simulink model "AttitudeControlPx4v1_8"  (R2018b)
settings: Solver=VariableStepAuto  StartTime=0.0  StopTime=10.0  RelTol=1e-3
settings Model: Creator=jban039  LastModifiedBy=jeremie

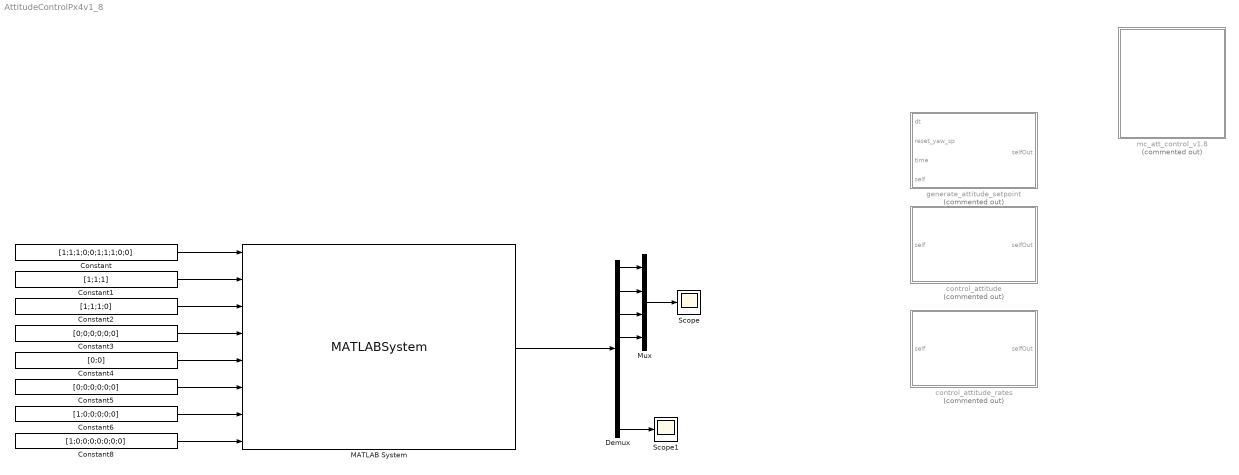
== system AttitudeControlPx4v1_8 ==
  Constant : Constant  Value=[1;1;1;0;0;1;1;1;0;0]
  Constant1 : Constant  Value=[1;1;1]
  Constant2 : Constant  Value=[1;1;1;0]
  Constant3 : Constant  Value=[0;0;0;0;0;0]
  Constant4 : Constant  Value=[0;0]
  Constant5 : Constant  Value=[0;0;0;0;0;0]
  Constant6 : Constant  Value=[1;0;0;0;0;0]
  Constant8 : Constant  Value=[1;0;0;0;0;0;0;0]
  Demux : Demux  Outputs=8
  MATLAB System : MATLABSystem  System=mc_att_control  acro_expo_rp=0.69  acro_expo_y=0.69  acro_pitch_max=720  acro_roll_max=720  acro_superexpo_rp=0.7  acro_superexpo_y=0.7  acro_yaw_max=540  airmode=0  d_term_cutoff_freq=30  pitch_rate_d=0.003  pitch_rate_ff=0  pitch_rate_i=0.05  pitch_rate_max=220  pitch_rate_p=0.15  pitch_p=6.5  pitch_rate_integ_lim=0.3  rattitude_thres=0.8  roll_rate_d=0.003  roll_rate_ff=0  roll_rate_i=0.05  roll_rate_max=220  roll_rate_p=0.15  roll_p=6.5  roll_rate_integ_lim=0.3  tpa_breakpoint_d=1  tpa_breakpoint_i=1  tpa_breakpoint_p=1  tpa_rate_d=0  tpa_rate_i=0  tpa_rate_p=0  yaw_rate_d=0  yaw_rate_ff=0  yaw_rate_i=0.1  yaw_rate_max=200  yaw_rate_p=0.2  yaw_auto_max=45  yaw_p=2.8  yaw_rate_integ_lim=0.3  man_throttle_min=0.08  man_tilt_max_deg=35  yaw_rate_scaling=200  throttle_hover=0.5  throttle_max=1  board_rotation_param=0  board_offset_x=0  board_offset_y=0  board_offset_z=0  bat_scale_en=0  throttle_curve=0  vehicle_status_is_rotary_wing=1  vehicle_status_is_vtol=0  loop_update_rate_hz=250  SimulateUsing=Code generation
      mask Type: mc_att_control
      mask Display:
      | disp(['mc_att_control' char(10) 'v1.8']);
      | port_label('input',1,'v_control_mode_flags');
      | port_label('input',2,'sensor_gyro');
      | port_label('input',3,'manual_control_sp_in');
      | port_label('input',4,'v_rates_sp_in');
      | port_label('input',5,'vehicle_land_detected_in');
      | port_label('input',6,'saturation_status_in');
      | port_label('input',7,'v_att_in');
      | port_label('input',8,'v_att_sp_in');
      | port_label('output',1,'actuators_control');
  Mux : Mux
  Scope : Scope
  Scope1 : Scope
  control_attitude : MATLAB Function  Commented=on  TreatAsAtomicUnit=on
  control_attitude_rates : MATLAB Function  Commented=on  TreatAsAtomicUnit=on
  generate_attitude_setpoint : MATLAB Function  Commented=on  TreatAsAtomicUnit=on
  mc_att_control_v1.8 : Subsystem  Commented=on
  wires:
  Constant/1 -> MATLAB System/1
  Constant8/1 -> MATLAB System/8
  Constant6/1 -> MATLAB System/7
  Constant1/1 -> MATLAB System/2
  Constant2/1 -> MATLAB System/3
  Constant3/1 -> MATLAB System/4
  Constant4/1 -> MATLAB System/5
  Constant5/1 -> MATLAB System/6
  MATLAB System/1 -> Demux/1
  Demux/1 -> Mux/1
  Demux/3 -> Mux/3
  Demux/4 -> Mux/4
  Demux/2 -> Mux/2
  Mux/1 -> Scope/1
  Demux/8 -> Scope1/1

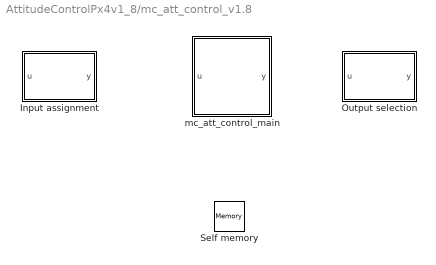
== system AttitudeControlPx4v1_8/mc_att_control_v1.8 ==
  Input assignment : MATLAB Function  TreatAsAtomicUnit=on
  Output selection : MATLAB Function  TreatAsAtomicUnit=on
  Self memory : Memory
  mc_att_control_main : MATLAB Function  TreatAsAtomicUnit=on

== matlab function AttitudeControlPx4v1_8/generate_attitude_setpoint ==
  data: dt input; selfOut output; reset_yaw_sp input; time input; self input
function selfOut =  generate_attitude_setpoint(dt, reset_yaw_sp, time, self)
%GENERATE_ATTITUDE_SETPOINT Generate attitude setpoint (manual control)
%   Based on code from PX4 Firmware (retrieved 2019/01/15, v1.82):
%       https://github.com/PX4/Firmware/blob/master/src/modules/mc_att_control/mc_att_control_main.cpp
%   Written:       J.X.J. Bannwarth, 2019/01/15
%   Last modified: J.X.J. Bannwarth, 2019/01/15

    eul = QuatToEuler( self.v_att.q );
    yaw = eul(3);
    if reset_yaw_sp
        self.man_yaw_sp = yaw;
    elseif ( self.manual_control_sp.z > 0.05 || strcmp( self.airmode, 'roll_pitch_yaw' ) )
        yaw_rate = self.yaw_rate_scaling;
        attitude_setpoint.yaw_sp_move_rate = self.manula_control_sp.r * yaw_rate;
        self.man_yaw_sp = wrap_pi( self.man_yaw_sp + attitude_setpoint.yaw_sp_move_rate*dt );
    end

    % Input mapping for roll & pitch setpoints
    % ----------------------------------------
    % We control the following 2 angles:
    % - tilt angle, given by sqrt(x*x + y*y)
    % - the direction of the maximum tilt in the XY-plane, which also
    % defines the direction of the motion
    %
    % This allows a simple limitation of the tilt angle, the vehicle flies
    % towards the direction that the stick points to, and changes of the
    % stick input are linear.
    x = self.manual_control_sp.x * self.man_tilt_max;
    y = self.manual_control_sp.y * self.man_tilt_max;
    
    % We want to fly towards the direction of (x, y), so we use a
    % perpendicular axis angle vector in the XY-plane
    v = [y, -x];
    v_norm = norm( v );
    
    if (v_norm > self.man_tilt_max) % limit to the configured maximum tilt angle
		v = v * self.man_tilt_max / v_norm;
    end
    
    q_sp_rpy = AxisAngleToQuat( [ v(1); v(2) ] );
    euler_sp = QuatToEuler( q_sp_rpy );
    attitude_setpoint.roll_body  = euler_sp(1);
    attitude_setpoint.pitch_body = euler_sp(2);
    % The axis angle can change the yaw as well (noticeable at higher tilt angles).
	% This is the formula by how much the yaw changes:
	%   let a := tilt angle, b := atan(y/x) (direction of maximum tilt)
	%   yaw = atan(-2 * sin(b) * cos(b) * sin^2(a/2) / (1 - 2 * cos^2(b) * sin^2(a/2))).
    attitude_setpoint.yaw_body = self.man_yaw_sp + euler_sp(3);
    
    if self.vehicle_status.is_vtol
        % Construct attitude setpoint rotation matrix. Modify the setpoints
        % for roll and pitch such that they reflect the user's intention
        % even if a large yaw error (yaw_sp - yaw) is present. In the
        % presence of a yaw error constructing a rotation matrix from the
        % pure euler angle setpoints will lead to unexpected attitude
        % behaviour from the user's view as the euler angle sequence uses
        % the  yaw setpoint and not the current heading of the vehicle.
		% However there's also a coupling effect that causes oscillations
        % for fast roll/pitch changes at higher tilt angles, so we want to
        % avoid using this on multicopters.
		% The effect of that can be seen with:
		% - roll/pitch into one direction, keep it fixed (at high angle)
		% - apply a fast yaw rotation
		% - look at the roll and pitch angles: they should stay pretty much
        % the same as when not yawing
        
        % Calculate our current yaw error
        yaw_error = wrap_pi(attitude_setpoint.yaw_body - yaw);

        % Compute the vector obtained by rotating a z unit vector by the rotation
        % given by the roll and pitch commands of the user
        zB = [0.0; 0.0; 1.0];
        R_sp_roll_pitch = EulerToDcm( [attitude_setpoint.roll_body; attitude_setpoint.pitch_body; 0.0] );
        z_roll_pitch_sp = R_sp_roll_pitch * zB;

        % Transform the vector into a new frame which is rotated around the z axis
        % by the current yaw error. this vector defines the desired tilt when we look
        % into the direction of the desired heading
        R_yaw_correction = EulerToDcm( [0.0; 0.0; -yaw_error] );
        z_roll_pitch_sp = R_yaw_correction * z_roll_pitch_sp;

        % Use the formula z_roll_pitch_sp = R_tilt * [0;0;1]
        % R_tilt is computed from_euler; only true if cos(roll) not equal zero
        % -> valid if roll is not +-pi/2;
        attitude_setpoint.roll_body = -asinf(z_roll_pitch_sp(1));
        attitude_setpoint.pitch_body = atan2f(z_roll_pitch_sp(0), z_roll_pitch_sp(2));
    end
    
    % Publish the setpoint
    q_sp = EulerToQuat( [ attitude_setpoint.roll_body;
                          attitude_setpoint.pitch_body;
                          attitude_setpoint.yaw_body ] );
    attitude_setpoint.q_d = q_sp;
    attitude_setpoint.q_d_valid = true;
    
    attitude_setpoint.thrust_body(3) = -throttle_curve( self.manual_control_sp.z );
    attitude_setpoint.timestamp = time;
end

% Other functions
function throttle = throttle_curve( throttle_stick_input, self )
    switch self.throttle_curve
        case 1 % no rescaling to hover throttle
            throttle = self.man_throttle_min + ...
                throttle_stick_input * (self.throttle_max - self.man_throttle_min);
        otherwise % 0 or other: rescale to hover throttle at 0.5 stick
            if throttle_stick_input < 0.5
                throttle = (self.throttle_hover - self.man_throttle_min) / ...
                    0.5 * throttle_stick_input + self.man_throttle_min;
            else
                throttle = (self.throttle_max - self.throttle_hover) / ...
                    0.5 * (throttle_stick_input - 1.0) + self.throttle_max;
            end
    end
end

% Angle functions
function euler = QuatToEuler( quat )
    euler = DcmToEuler( QuatToDcm( quat ) );
end

function euler = DcmToEuler( dcm )
%DCMTOEULER Convert DCM to Euler angles
%   Based on code from PX4 Firmware:
%       https://github.com/PX4/Matrix/blob/master/matrix/Euler.hpp
%   Written:       J.X.J. Bannwarth, 2019/01/15
%   Last modified: J.X.J. Bannwarth, 2019/01/15
    phi_val   = atan2( dcm(3,2), dcm(3,3) );
    theta_val = asin( -dcm(3,1) );
    psi_val   = atan2( dcm(2,1), dcm(1,1) );
    if abs( theta_val - pi/2 ) < 1e-3
        phi_val = 0;
        psi_val = atan2( dcm(2,3), dcm(1,3) );
    elseif abs( theta_val + pi /2 ) < 1e-3
        phi_val = 0;
        psi_val = atan2( -dcm(2,3), -dcm(1,3) );
    end
    
    euler = [ phi_val; theta_val; psi_val ];
end

function dcm = QuatToDcm( quat )
%DCMTOEULER Convert quaternion to DCM
%   Based on code from PX4 Firmware:
%       https://github.com/PX4/Matrix/blob/master/matrix/Dcm.hpp
%   Written:       J.X.J. Bannwarth, 2019/01/15
%   Last modified: J.X.J. Bannwarth, 2019/01/15
    a = quat(1);
    b = quat(2);
    c = quat(3);
    d = quat(4);
    aa = a * a;
    ab = a * b;
    ac = a * c;
    ad = a * d;
    bb = b * b;
    bc = b * c;
    bd = b * d;
    cc = c * c;
    cd = c * d;
    dd = d * d;

    dcm = zeros(3, 3);
    dcm(1, 1) = aa + bb - cc - dd;
    dcm(1, 2) = 2 * (bc - ad);
    dcm(1, 3) = 2 * (ac + bd);
    dcm(2, 1) = 2 * (bc + ad);
    dcm(2, 2) = aa - bb + cc - dd;
    dcm(2, 3) = 2 * (cd - ab);
    dcm(3, 1) = 2 * (bd - ac);
    dcm(3, 2) = 2 * (ab + cd);
    dcm(3, 3) = aa - bb - cc + dd;
end

function dcm = EulerToDcm( eul )
%EULERTODCM Convert Euler angles to a DCM
%   Based on code from PX4 Firmware:
%       https://github.com/PX4/Matrix/blob/master/matrix/Dcm.hpp
%   Written:       J.X.J. Bannwarth, 2019/01/15
%   Last modified: J.X.J. Bannwarth, 2019/01/15
    phi   = eul(1);
    theta = eul(2);
    psi   = eul(3);
    sinPhi = sin(phi);
    cosPhi = cos(phi);
    cosThe = cos(theta);
    sinThe = sin(theta);
    sinPsi = sin(psi);
    cosPsi = cos(psi);
    
    dcm = zeros(3,3);
    dcm(1,1) = cosThe * cosPsi;
    dcm(1,2) = (sinPhi * sinThe * cosPsi) - (cosPhi * sinPsi);
    dcm(1,3) = (cosPhi * sinThe * cosPsi) + (sinPhi * sinPsi);
    dcm(2,1) = cosThe * sinPsi;
    dcm(2,2) = (sinPhi * sinThe * sinPsi) + (cosPhi * cosPsi);
    dcm(2,3) = (cosPhi * sinThe * sinPsi) - (sinPhi * cosPsi);
    dcm(3,1) = -sinThe;
    dcm(3,2) = sinPhi * cosThe;
    dcm(3,3) = cosPhi * cosThe;
end

function quat = AxisAngleToQuat( axisAngle )
%AXISANGLETOQUAT Convert axis angle representation to quaternion
%   Based on code from PX4 Firmware:
%       https://github.com/PX4/Matrix/blob/master/matrix/Quaternion.hpp
%   axisAngle = [x; y; z]*angle where [x; y; z] is a unit vector
%   Written:       J.X.J. Bannwarth, 2019/01/15
%   Last modified: J.X.J. Bannwarth, 2019/01/15

    angle = norm(axisAngle);
    axis = axisAngle / angle;
    quat = zeros(4,1);
    if (angle < 1e-10)
        quat(1) = 1.0;
        % quat(1) = quat(2) = quat(3) = 0;
    else
        magnitude = sin(angle / 2.0);
        quat(1) = cos(angle / 2.0);
        quat(2) = axis(1) * magnitude;
        quat(3) = axis(2) * magnitude;
        quat(4) = axis(3) * magnitude;
    end
end

function bearing = wrap_pi(bearing)
    % value is inf or NaN
    if (~isfinite(bearing))
        bearing = nan;
        return
    end

    c = 0;

    while (bearing >= 3.14159265)
        bearing = bearing - 6.28318531;

        if (c > 3)
            bearing = nan;
            return
        end
        c = c + 1;
    end

    c = 0;

    while (bearing < -3.14159265)
        bearing = bearing + 6.28318531;

        if (c > 3)
            bearing = nan;
            return
        end
        c = c + 1;
    end
end

== matlab function AttitudeControlPx4v1_8/control_attitude ==
  data: selfOut output; self input
function selfOut =  control_attitude( self )
%CONTROL_ATTITUDE Attitude controller
%   Based on code from PX4 Firmware (retrieved 2019/01/15, v1.82):
%       https://github.com/PX4/Firmware/blob/master/src/modules/mc_att_control/mc_att_control_main.cpp
%   Input: 'vehicle_attitude_setpoint' (depending on mode)
%   Output: self.rates_sp, self.thrust_sp
%   Written:       J.X.J. Bannwarth, 2019/01/15
%   Last modified: J.X.J. Bannwarth, 2019/01/15

    % Physical thrust axis is the negative of body z axis
    self.thrust_sp = -self.v_att_sp.thrust_body(3);

    % Prepare yaw weight from the ratio between roll/pitch and yaw gains
    attitude_gain = self.attitude_p;
    roll_pitch_gain = ( attitude_gain(1) + attitude_gain(2) ) / 2;
    yaw_w = constrain( attitude_gain(3) / roll_pitch_gain, 0, 1 );
    attitude_gain(2) = roll_pitch_gain;

    % Get estimated and desired vehicle attitude
    q  = self.v_att.q;
    qd = self.v_att_sp.q_d;

    % Ensure input quaternions are exactly normalized because
    % acosf(1.00001) == NaN
    q = normalize( q );
    qd = normalize( qd );

    % Calculate reduced desired attitude neglecting vehicle's yaw to
    % prioritize roll and pitch 
    e_z   = QuatToDcmZ( q );
    e_z_d = QuatToDcmZ( qd );
    qd_red = VecsToQuat( e_z, e_z_d );
    
    if ( abs(qd_red(2)) > (1 - 1e-5) ) || ( abs(qd_red(3)) > (1 - 1e-5) )
        % In the infinitesimal corner case where the vehicle and thrust have
        % the completely opposite direction, full attitude control anyways
        % generates no yaw input and directly takes the combination of roll
        % and pitch leading to the correct desired yaw. Ignoring this case
        % would still be totally safe and stable.
        qd_red = qd;
    else
        % Transform rotation from current to desired thrust vector into a
        % world frame reduced desired attitude
        qd_red = qd_red * q;
    end
    
    % Mix full and reduced desired attitude
    q_mix = QuatMult( InvertQuat(qd_red), qd );
    q_mix = q_mix * SignNoZero( q_mix(1) );
    
    % Catch numerical problems with the domain of acosf and asinf
    q_mix(1) = constrain( q_mix(1), -1, 1 );
    q_mix(4) = constrain( q_mix(4), -1, 1 );
    qd = qd_red * [ cos( yaw_w * acos(q_mix(1)) );
                    0;
                    0;
                    sin( yaw_w * asin(q_mix(4)) ) ];

    % Quaternion attitude control law, qe is rotation from q to qd
    qe = QuatMult( InvertQuat(q), qd );

    % Using sin(alpha/2) scaled rotation axis as attitude error (see
    % quaternion definition by axis angle)
    % Also taking care of the antipodal unit quaternion ambiguity
    % qe(2:4) corresponds to the imaginary part of the quaternion
    eq = 2 .* SignNoZero(qe(1)) .* qe(2:4);

    % calculate angular rates setpoint
    self.rates_sp = eq .* attitude_gain;

    % Feed forward the yaw setpoint rate.
    % yaw_sp_move_rate is the feed forward commanded rotation around the
    % world z-axis, but we need to apply it in the body frame (because
    % self.rates_sp is expressed in the body frame).
    % Therefore we infer the world z-axis (expressed in the body frame) by
    % taking the last column of R.transposed (== q.inversed) and multiply
    % it by the yaw setpoint rate (yaw_sp_move_rate).
    % This yields a vector representing the commanded rotation around the
    % world z-axis expressed in the body frame such that it can be added to
    % the rates setpoint.
    self.rates_sp = self.rates_sp + QuatToDcmZ( InvertQuat(q) ) * self.v_att_sp.yaw_sp_move_rate;
    
    % limit rates
    for i = 1:3
        if (( self.v_control_mode.flag_control_velocity_enabled || ...
                self.v_control_mode.flag_control_auto_enabled ) && ...
                ~self.v_control_mode.flag_control_manual_enabled )
            self.rates_sp(i) = constrain(self.rates_sp(i), -self.auto_rate_max(i), self.auto_rate_max(i));
        else
            self.rates_sp(i) = constrain(self.rates_sp(i), -self.mc_rate_max(i), self.mc_rate_max(i));
        end
    end
end

% Other functions
function out = normalize( in )
    out = in ./ norm(in);
end

function y = constrain( x, x_min, x_max )
    y = max( min(x, x_max), x_min );
end

function out = SignNoZero( in )
%SIGNNOZERO SIGNUM function that returns 1 at 0
%   Based on code from PX4 Firmware:
%       https://github.com/PX4/Firmware/blob/master/src/lib/mathlib/math/Functions.hpp
%   Written:       J.X.J. Bannwarth, 2019/01/15
%   Last modified: J.X.J. Bannwarth, 2019/01/17
    out = ( 0 <= in ) - ( in < 0 );
end

% Angle functions
function euler = QuatToEuler( quat )
    euler = DcmToEuler( QuatToDcm( quat ) );
end

function euler = DcmToEuler( dcm )
%DCMTOEULER Convert DCM to Euler angles
%   Based on code from PX4 Firmware:
%       https://github.com/PX4/Matrix/blob/master/matrix/Euler.hpp
%   Written:       J.X.J. Bannwarth, 2019/01/15
%   Last modified: J.X.J. Bannwarth, 2019/01/15
    phi_val   = atan2( dcm(3,2), dcm(3,3) );
    theta_val = asin( -dcm(3,1) );
    psi_val   = atan2( dcm(2,1), dcm(1,1) );
    if abs( theta_val - pi/2 ) < 1e-3
        phi_val = 0;
        psi_val = atan2( dcm(2,3), dcm(1,3) );
    elseif abs( theta_val + pi /2 ) < 1e-3
        phi_val = 0;
        psi_val = atan2( -dcm(2,3), -dcm(1,3) );
    end
    
    euler = [ phi_val; theta_val; psi_val ];
end

function dcm = QuatToDcm( quat )
%QUATTODCM Convert quaternion to DCM
%   Based on code from PX4 Firmware:
%       https://github.com/PX4/Matrix/blob/master/matrix/Dcm.hpp
%   Written:       J.X.J. Bannwarth, 2019/01/15
%   Last modified: J.X.J. Bannwarth, 2019/01/15
    a = quat(1);
    b = quat(2);
    c = quat(3);
    d = quat(4);
    aa = a * a;
    ab = a * b;
    ac = a * c;
    ad = a * d;
    bb = b * b;
    bc = b * c;
    bd = b * d;
    cc = c * c;
    cd = c * d;
    dd = d * d;

    dcm = zeros(3, 3);
    dcm(1, 1) = aa + bb - cc - dd;
    dcm(1, 2) = 2 * (bc - ad);
    dcm(1, 3) = 2 * (ac + bd);
    dcm(2, 1) = 2 * (bc + ad);
    dcm(2, 2) = aa - bb + cc - dd;
    dcm(2, 3) = 2 * (cd - ab);
    dcm(3, 1) = 2 * (bd - ac);
    dcm(3, 2) = 2 * (ab + cd);
    dcm(3, 3) = aa - bb - cc + dd;
end

function dcmZ = QuatToDcmZ( quat )
%QUATTODCMZ Convert quaternion to corresponding body z-axis
%	Last orthogonal unit basis vector
%   == last column of the equivalent rotation matrix
%   but calculated more efficiently than a full conversion
%   Based on code from PX4 Firmware:
%       https://github.com/PX4/Matrix/blob/master/matrix/Dcm.hpp
%   Written:       J.X.J. Bannwarth, 2019/01/15
%   Last modified: J.X.J. Bannwarth, 2019/01/15

    a = quat(1);
    b = quat(2);
    c = quat(3);
    d = quat(4);
    dcmZ = [ 2 * (a * c + b * d);
             2 * (c * d - a * b);
             a * a - b * b - c * c + d * d ];
end

function dcm = EulerToDcm( eul )
%EULERTODCM Convert Euler angles to a DCM
%   Based on code from PX4 Firmware:
%       https://github.com/PX4/Matrix/blob/master/matrix/Dcm.hpp
%   Written:       J.X.J. Bannwarth, 2019/01/15
%   Last modified: J.X.J. Bannwarth, 2019/01/15
    phi   = eul(1);
    theta = eul(2);
    psi   = eul(3);
    sinPhi = sin(phi);
    cosPhi = cos(phi);
    cosThe = cos(theta);
    sinThe = sin(theta);
    sinPsi = sin(psi);
    cosPsi = cos(psi);
    
    dcm = zeros(3,3);
    dcm(1,1) = cosThe * cosPsi;
    dcm(1,2) = (sinPhi * sinThe * cosPsi) - (cosPhi * sinPsi);
    dcm(1,3) = (cosPhi * sinThe * cosPsi) + (sinPhi * sinPsi);
    dcm(2,1) = cosThe * sinPsi;
    dcm(2,2) = (sinPhi * sinThe * sinPsi) + (cosPhi * cosPsi);
    dcm(2,3) = (cosPhi * sinThe * sinPsi) - (sinPhi * cosPsi);
    dcm(3,1) = -sinThe;
    dcm(3,2) = sinPhi * cosThe;
    dcm(3,3) = cosPhi * cosThe;
end

function quat = AxisAngleToQuat( axisAngle )
%AXISANGLETOQUAT Convert axis angle representation to quaternion
%   axisAngle = [x; y; z]*angle where [x; y; z] is a unit vector
%   Based on code from PX4 Firmware:
%       https://github.com/PX4/Matrix/blob/master/matrix/Quaternion.hpp
%   Written:       J.X.J. Bannwarth, 2019/01/15
%   Last modified: J.X.J. Bannwarth, 2019/01/15

    angle = norm(axisAngle);
    axis = axisAngle / angle;
    quat = zeros(4,1);
    if (angle < 1e-10)
        quat(1) = 1.0;
        % quat(1) = quat(2) = quat(3) = 0;
    else
        magnitude = sin(angle / 2.0);
        quat(1) = cos(angle / 2.0);
        quat(2) = axis(1) * magnitude;
        quat(3) = axis(2) * magnitude;
        quat(4) = axis(3) * magnitude;
    end
end

function quat = VecsToQuat( src, dst )
%VECSTOQUAT Quaternion from two vectors
%   Generates shortest rotation from source to destination vector
%   Based on code from PX4 Firmware:
%       https://github.com/PX4/Matrix/blob/master/matrix/Quaternion.hpp
%   Written:       J.X.J. Bannwarth, 2019/01/15
%   Last modified: J.X.J. Bannwarth, 2019/01/15
    cr = cross(src, dst);
    dt = dot(src, dst);
    quat = zeros(4,1);
    locEps = 1e-5; % Don't use eps as it's a reserved variable in MATLAB
    if (norm(cr) < locEps && dt < 0)
        % Handle corner cases with 180 degree rotations
        % If the two vectors are parallel, cross product is zero
        % If they point opposite, the dot product is negative
        cr = abs(src);
        if (cr(1) < cr(2))
            if (cr(1) < cr(3))
                cr = [1; 0; 0];
            else
                cr = [0; 0; 1];
            end
        else
            if (cr(2) < cr(3))
                cr = [0; 1; 0];
            else
                cr = [0; 0; 1];
            end
        end
        quat(1) = 0;
        cr = cross(src, cr);
    else
        % Normal case, do half-way quaternion solution
        quat(1) = dt + sqrt( norm(src)^2 * norm(dst)^2 );
    end
    quat(2) = cr(1);
    quat(3) = cr(2);
    quat(4) = cr(3);
    quat = normalize( quat );
end

function quatInv = InvertQuat( quat )
%INVERTQUAT Invert quaternion
%   Based on code from PX4 Firmware:
%       https://github.com/PX4/Matrix/blob/master/matrix/Quaternion.hpp
%   Written:       J.X.J. Bannwarth, 2019/01/15
%   Last modified: J.X.J. Bannwarth, 2019/01/15
    normSq = dot( quat, quat );
    quatInv = ( quat .* [1;-1;-1;-1] ./ normSq );
end

function quatOut = QuatMult( q1, q2 )
%QUATMULT Multiply quaternion q1 by quaternion q2
%   Based on code from PX4 Firmware:
%       https://github.com/PX4/Matrix/blob/master/matrix/Quaternion.hpp
%   Written by:    J.X.J. Bannwarth, 2017/03/28
%   Last modified: J.X.J. Bannwarth, 2017/01/15
    quatOut = [ q1(1) * q2(1) - q1(2) * q2(2) - q1(3) * q2(3) - q1(4) * q2(4) ;
                q1(1) * q2(2) + q1(2) * q2(1) + q1(3) * q2(4) - q1(4) * q2(3) ;
                q1(1) * q2(3) - q1(2) * q2(4) + q1(3) * q2(1) + q1(4) * q2(2) ;
                q1(1) * q2(4) + q1(2) * q2(3) - q1(3) * q2(2) + q1(4) * q2(1) ];
end

function bearing = wrap_pi(bearing)
    % value is inf or NaN
    if (~isfinite(bearing))
        bearing = nan;
        return
    end

    c = 0;

    while (bearing >= 3.14159265)
        bearing = bearing - 6.28318531;

        if (c > 3)
            bearing = nan;
            return
        end
        c = c + 1;
    end

    c = 0;

    while (bearing < -3.14159265)
        bearing = bearing + 6.28318531;

        if (c > 3)
            bearing = nan;
            return
        end
        c = c + 1;
    end
end

== matlab function AttitudeControlPx4v1_8/control_attitude_rates ==
  data: selfOut output; self input
function selfOut =  control_attitude_rates( self )
%CONTROL_ATTITUDE_RATES Attitude rates controller
%   Based on code from PX4 Firmware (retrieved 2019/01/15, v1.82):
%       https://github.com/PX4/Firmware/blob/master/src/modules/mc_att_control/mc_att_control_main.cpp
%   Input: self.rates_sp, self.thrust_sp
%   Output: self.att_control
%   Written:       J.X.J. Bannwarth, 2019/01/15
%   Last modified: J.X.J. Bannwarth, 2019/01/16

    % Reset integral if disarmed */
    if (~self.v_control_mode.flag_armed || self.vehicle_status.is_rotary_wing)
        self.rates_int = zeros(3,1);
    end

    % Get the raw gyro data and correct for thermal errors
    % Note: the original code applies different correction based on which
    % gyro is being used, but since this is a simulation we do not need to
    % worry about this.
    rates = zeros(3,1);
    rates(1) = self.sensor_gyro.x;
    rates(2) = self.sensor_gyro.y;
    rates(3) = self.sensor_gyro.z;

    % Rotate corrected measurements from sensor to body frame
    rates = self.board_rotation * rates;

    % Correct for in-run bias errors
    rates(1) = rates(1) - self.sensor_bias.gyro_x_bias;
    rates(2) = rates(2) - self.sensor_bias.gyro_y_bias;
    rates(3) = rates(3) - self.sensor_bias.gyro_z_bias;

    rates_p_scaled = self.rate_p .* pid_attenuations(self.tpa_breakpoint_p, self.tpa_rate_p, self.thrust_sp);
    rates_i_scaled = self.rate_i .* pid_attenuations(self.tpa_breakpoint_i, self.tpa_rate_i, self.thrust_sp);
    rates_d_scaled = self.rate_d .* pid_attenuations(self.tpa_breakpoint_d, self.tpa_rate_d, self.thrust_sp);

    % Angular rates error
    rates_err = self.rates_sp - rates;

    % Apply low-pass filtering to the rates for D-term
    [ rates_filtered, self.lp_filters_d ] = LowPassFilter2pVector3Apply( rates, self.lp_filters_d );

    self.att_control = rates_p_scaled .* rates_err + ...
        self.rates_int - ...
        rates_d_scaled .* (rates_filtered - self.rates_prev_filtered) / dt + ...
        self.rate_ff .* self.rates_sp;

    self.rates_prev = rates;
    self.rates_prev_filtered = rates_filtered;

    % update integral only if we are not landed */
    if (~self.vehicle_land_detected.maybe_landed && ~self.vehicle_land_detected.landed)
        for i = 1:3
            % Check for positive control saturation
            positive_saturation = ...
                ((i == 1) && self.saturation_status.flags.roll_pos) || ...
                ((i == 2) && self.saturation_status.flags.pitch_pos) || ...
                ((i == 3) && self.saturation_status.flags.yaw_pos);

            % Check for negative control saturation
            negative_saturation = ...
                ((i == 1) && self.saturation_status.flags.roll_neg) || ...
                ((i == 2) && self.saturation_status.flags.pitch_neg) || ...
                ((i == 3) && self.saturation_status.flags.yaw_neg);

            % prevent further positive control saturation
            if (positive_saturation)
                rates_err(i) = min( [rates_err(i), 0.0] );
            end

            % prevent further negative control saturation
            if (negative_saturation)
                rates_err(i) = max( [rates_err(i), 0.0] );
            end

            % Perform the integration using a first order method and do not propagate the result if out of range or invalid
            rate_i = self.rates_int(i) + rates_i_scaled(i) * rates_err(i) * dt;

            if (isfinite(rate_i) && (rate_i > -self.rate_int_lim(i)) && (rate_i < self.rate_int_lim(i)))
                self.rates_int(i) = rate_i;
            end
        end
    end

    % explicitly limit the integrator state */
    for i = 1:3
        self.rates_int(i) = constrain(self.rates_int(i), -self.rate_int_lim(i), self.rate_int_lim(i));
    end

end

% Other functions
function out = normalize( in )
    out = in ./ norm(in);
end

function y = constrain( x, x_min, x_max )
    y = max( min(x, x_max), x_min );
end

function out = SignNoZero( in )
%SIGNNOZERO SIGNUM function that returns 1 at 0
%   Based on code from PX4 Firmware:
%       https://github.com/PX4/Firmware/blob/master/src/lib/mathlib/math/Functions.hpp
%   Written:       J.X.J. Bannwarth, 2019/01/15
%   Last modified: J.X.J. Bannwarth, 2019/01/17
    out = ( 0 <= in ) - ( in < 0 );
end

function pidAttenuationPerAxis = pid_attenuations( tpa_breakpoint, tpa_rate, thrust_sp )
%PID_ATTENUATIONS Throttle PID attenuation
%   Function visualization available here https://www.desmos.com/calculator/gn4mfoddje
%   Input: tpa_breakpoint, tpa_rate, self.thrust_sp
%   Based on code from PX4 Firmware:
%       https://github.com/PX4/Firmware/blob/master/src/modules/mc_att_control/mc_att_control_main.cpp
%   Written:       J.X.J. Bannwarth, 2019/01/16
%   Last modified: J.X.J. Bannwarth, 2019/01/16
    TPA_RATE_LOWER_LIMIT = 0.05;
    tpa = 1.0 - tpa_rate * (abs(thrust_sp) - tpa_breakpoint) / (1.0 - tpa_breakpoint);
    tpa = max([TPA_RATE_LOWER_LIMIT, min([1.0, tpa])]);
    pidAttenuationPerAxis = [ tpa; tpa; 1.0 ];
end

% Lowpass
function [ output, filter ] = LowPassFilter2pVector3Apply( sample, filter )
%LOWPASSFILTER2PVECTOR3APPLY Apply low pass filter
%   Based on code from PX4 Firmware:
%       https://github.com/PX4/Firmware/blob/master/src/lib/mathlib/math/filter/LowPassFilter2pVector3f.hpp
%   Written:       J.X.J. Bannwarth, 2019/01/16
%   Last modified: J.X.J. Bannwarth, 2019/01/16
    delay_element_0 = sample - filter.delay_element_1.*filter.a1 - filter.delay_element_2.*filter.a2;
    output = delay_element_0.*filter.b0 + filter.delay_element_1.*filter.b1 + filter.delay_element_2*filter.b2;
    filter.delay_element_2 = filter.delay_element_1;
    filter.delay_element_1 = delay_element_0;
end

function filter = LowPassFilter2pVectorSetCutOffFrequency( sample_freq, cutoff_freq, filter )
%LOWPASSFILTER2PVECTOR3SETCUTOFFFREQUENCY Set cutoff frequency
%   Based on code from PX4 Firmware:
%       https://github.com/PX4/Firmware/blob/master/src/lib/mathlib/math/filter/LowPassFilter2pVector3f.cpp
%   Written:       J.X.J. Bannwarth, 2019/01/16
%   Last modified: J.X.J. Bannwarth, 2019/01/16
    filter.cutoff_freq = cutoff_freq;

    % Reset delay elements on filter change
    filter.delay_element_1 = zeros(3,1);
    filter.delay_element_2 = zeros(3,1);

    if (filter.cutoff_freq <= 0.0)
        % No filtering
        filter.b0 = 1.0;
        filter.b1 = 0.0;
        filter.b2 = 0.0;

        filter.a1 = 0.0;
        filter.a2 = 0.0;
        return
    end

    fr = sample_freq / filter.cutoff_freq;
    ohm = tanf( pi / fr);
    c = 1.0 + 2.0 * cosf( pi / 4.0) * ohm + ohm * ohm;

    filter.b0 = ohm * ohm / c;
    filter.b1 = 2.0 * filter.b0;
    filter.b2 = filter.b0;

    filter.a1 = 2.0 * (ohm * ohm - 1.0) / c;
    filter.a2 = (1.0 - 2.0 * cosf(pi / 4.0) * ohm + ohm * ohm) / c;
end

function [ output, filter ] = LowPassFilter2pVectorReset( sample, filter )
%LOWPASSFILTER2PVECTOR3SETCUTOFFFREQUENCY Set cutoff frequency
%   Based on code from PX4 Firmware:
%       https://github.com/PX4/Firmware/blob/master/src/lib/mathlib/math/filter/LowPassFilter2pVector3f.cpp
%   Written:       J.X.J. Bannwarth, 2019/01/16
%   Last modified: J.X.J. Bannwarth, 2019/01/16
    dval = sample ./ (filter.b0 + filter.b1 + filter.b2);

    if (isfinite( dval(1) ) && isfinite( dval(2) ) && isfinite( dval(3) ))
        filter.delay_element_1 = dval;
        filter.delay_element_2 = dval;
    else
        filter.delay_element_1 = sample;
        filter.delay_element_2 = sample;
    end

    [ output, filter ] = LowPassFilter2pVector3Apply( sample, filter );
end

% Angle functions  
function euler = QuatToEuler( quat )
    euler = DcmToEuler( QuatToDcm( quat ) );
end

function euler = DcmToEuler( dcm )
%DCMTOEULER Convert DCM to Euler angles
%   Based on code from PX4 Firmware:
%       https://github.com/PX4/Matrix/blob/master/matrix/Euler.hpp
%   Written:       J.X.J. Bannwarth, 2019/01/15
%   Last modified: J.X.J. Bannwarth, 2019/01/15
    phi_val   = atan2( dcm(3,2), dcm(3,3) );
    theta_val = asin( -dcm(3,1) );
    psi_val   = atan2( dcm(2,1), dcm(1,1) );
    if abs( theta_val - pi/2 ) < 1e-3
        phi_val = 0;
        psi_val = atan2( dcm(2,3), dcm(1,3) );
    elseif abs( theta_val + pi /2 ) < 1e-3
        phi_val = 0;
        psi_val = atan2( -dcm(2,3), -dcm(1,3) );
    end
    
    euler = [ phi_val; theta_val; psi_val ];
end

function dcm = QuatToDcm( quat )
%QUATTODCM Convert quaternion to DCM
%   Based on code from PX4 Firmware:
%       https://github.com/PX4/Matrix/blob/master/matrix/Dcm.hpp
%   Written:       J.X.J. Bannwarth, 2019/01/15
%   Last modified: J.X.J. Bannwarth, 2019/01/15
    a = quat(1);
    b = quat(2);
    c = quat(3);
    d = quat(4);
    aa = a * a;
    ab = a * b;
    ac = a * c;
    ad = a * d;
    bb = b * b;
    bc = b * c;
    bd = b * d;
    cc = c * c;
    cd = c * d;
    dd = d * d;

    dcm = zeros(3, 3);
    dcm(1, 1) = aa + bb - cc - dd;
    dcm(1, 2) = 2 * (bc - ad);
    dcm(1, 3) = 2 * (ac + bd);
    dcm(2, 1) = 2 * (bc + ad);
    dcm(2, 2) = aa - bb + cc - dd;
    dcm(2, 3) = 2 * (cd - ab);
    dcm(3, 1) = 2 * (bd - ac);
    dcm(3, 2) = 2 * (ab + cd);
    dcm(3, 3) = aa - bb - cc + dd;
end

function dcmZ = QuatToDcmZ( quat )
%QUATTODCMZ Convert quaternion to corresponding body z-axis
%	Last orthogonal unit basis vector
%   == last column of the equivalent rotation matrix
%   but calculated more efficiently than a full conversion
%   Based on code from PX4 Firmware:
%       https://github.com/PX4/Matrix/blob/master/matrix/Dcm.hpp
%   Written:       J.X.J. Bannwarth, 2019/01/15
%   Last modified: J.X.J. Bannwarth, 2019/01/15

    a = quat(1);
    b = quat(2);
    c = quat(3);
    d = quat(4);
    dcmZ = [ 2 * (a * c + b * d);
             2 * (c * d - a * b);
             a * a - b * b - c * c + d * d ];
end

function dcm = EulerToDcm( eul )
%EULERTODCM Convert Euler angles to a DCM
%   Based on code from PX4 Firmware:
%       https://github.com/PX4/Matrix/blob/master/matrix/Dcm.hpp
%   Written:       J.X.J. Bannwarth, 2019/01/15
%   Last modified: J.X.J. Bannwarth, 2019/01/15
    phi   = eul(1);
    theta = eul(2);
    psi   = eul(3);
    sinPhi = sin(phi);
    cosPhi = cos(phi);
    cosThe = cos(theta);
    sinThe = sin(theta);
    sinPsi = sin(psi);
    cosPsi = cos(psi);
    
    dcm = zeros(3,3);
    dcm(1,1) = cosThe * cosPsi;
    dcm(1,2) = (sinPhi * sinThe * cosPsi) - (cosPhi * sinPsi);
    dcm(1,3) = (cosPhi * sinThe * cosPsi) + (sinPhi * sinPsi);
    dcm(2,1) = cosThe * sinPsi;
    dcm(2,2) = (sinPhi * sinThe * sinPsi) + (cosPhi * cosPsi);
    dcm(2,3) = (cosPhi * sinThe * sinPsi) - (sinPhi * cosPsi);
    dcm(3,1) = -sinThe;
    dcm(3,2) = sinPhi * cosThe;
    dcm(3,3) = cosPhi * cosThe;
end

function quat = AxisAngleToQuat( axisAngle )
%AXISANGLETOQUAT Convert axis angle representation to quaternion
%   axisAngle = [x; y; z]*angle where [x; y; z] is a unit vector
%   Based on code from PX4 Firmware:
%       https://github.com/PX4/Matrix/blob/master/matrix/Quaternion.hpp
%   Written:       J.X.J. Bannwarth, 2019/01/15
%   Last modified: J.X.J. Bannwarth, 2019/01/15

    angle = norm(axisAngle);
    axis = axisAngle / angle;
    quat = zeros(4,1);
    if (angle < 1e-10)
        quat(1) = 1.0;
        % quat(1) = quat(2) = quat(3) = 0;
    else
        magnitude = sin(angle / 2.0);
        quat(1) = cos(angle / 2.0);
        quat(2) = axis(1) * magnitude;
        quat(3) = axis(2) * magnitude;
        quat(4) = axis(3) * magnitude;
    end
end

function quat = VecsToQuat( src, dst )
%VECSTOQUAT Quaternion from two vectors
%   Generates shortest rotation from source to destination vector
%   Based on code from PX4 Firmware:
%       https://github.com/PX4/Matrix/blob/master/matrix/Quaternion.hpp
%   Written:       J.X.J. Bannwarth, 2019/01/15
%   Last modified: J.X.J. Bannwarth, 2019/01/15
    cr = cross(src, dst);
    dt = dot(src, dst);
    quat = zeros(4,1);
    locEps = 1e-5; % Don't use eps as it's a reserved variable in MATLAB
    if (norm(cr) < locEps && dt < 0)
        % Handle corner cases with 180 degree rotations
        % If the two vectors are parallel, cross product is zero
        % If they point opposite, the dot product is negative
        cr = abs(src);
        if (cr(1) < cr(2))
            if (cr(1) < cr(3))
                cr = [1; 0; 0];
            else
                cr = [0; 0; 1];
            end
        else
            if (cr(2) < cr(3))
                cr = [0; 1; 0];
            else
                cr = [0; 0; 1];
            end
        end
        quat(1) = 0;
        cr = cross(src, cr);
    else
        % Normal case, do half-way quaternion solution
        quat(1) = dt + sqrt( norm(src)^2 * norm(dst)^2 );
    end
    quat(2) = cr(1);
    quat(3) = cr(2);
    quat(4) = cr(3);
    quat = normalize( quat );
end

function quatInv = InvertQuat( quat )
%INVERTQUAT Invert quaternion
%   Based on code from PX4 Firmware:
%       https://github.com/PX4/Matrix/blob/master/matrix/Quaternion.hpp
%   Written:       J.X.J. Bannwarth, 2019/01/15
%   Last modified: J.X.J. Bannwarth, 2019/01/15
    normSq = dot( quat, quat );
    quatInv = ( quat .* [1;-1;-1;-1] ./ normSq );
end

function quatOut = QuatMult( q1, q2 )
%QUATMULT Multiply quaternion q1 by quaternion q2
%   Based on code from PX4 Firmware:
%       https://github.com/PX4/Matrix/blob/master/matrix/Quaternion.hpp
%   Written by:    J.X.J. Bannwarth, 2017/03/28
%   Last modified: J.X.J. Bannwarth, 2017/01/15
    quatOut = [ q1(1) * q2(1) - q1(2) * q2(2) - q1(3) * q2(3) - q1(4) * q2(4) ;
                q1(1) * q2(2) + q1(2) * q2(1) + q1(3) * q2(4) - q1(4) * q2(3) ;
                q1(1) * q2(3) - q1(2) * q2(4) + q1(3) * q2(1) + q1(4) * q2(2) ;
                q1(1) * q2(4) + q1(2) * q2(3) - q1(3) * q2(2) + q1(4) * q2(1) ];
end

function bearing = wrap_pi(bearing)
    % value is inf or NaN
    if (~isfinite(bearing))
        bearing = nan;
        return
    end

    c = 0;

    while (bearing >= 3.14159265)
        bearing = bearing - 6.28318531;

        if (c > 3)
            bearing = nan;
            return
        end
        c = c + 1;
    end

    c = 0;

    while (bearing < -3.14159265)
        bearing = bearing + 6.28318531;

        if (c > 3)
            bearing = nan;
            return
        end
        c = c + 1;
    end
end

== matlab function AttitudeControlPx4v1_8/mc_att_control_v1.8/Output selection ==
  data: u input; y output
function y = fcn(u)

y = u;

== matlab function AttitudeControlPx4v1_8/mc_att_control_v1.8/Input assignment ==
  data: u input; y output
function y = fcn(u)

y = u;

== matlab function AttitudeControlPx4v1_8/mc_att_control_v1.8/mc_att_control_main ==
  data: u input; y output
function y = fcn(u)

y = u;
